simulink model "FMtest"  (R2021a)
settings: Solver=VariableStepAuto  StartTime=0.0  StopTime=3  RelTol=1e-3
undefined symbols (not defined in the file or in its folder): National_Instruments, PCIe
libraries: sldrtlib x4
settings Model: Creator=simmo536  LastModifiedBy=simmo536

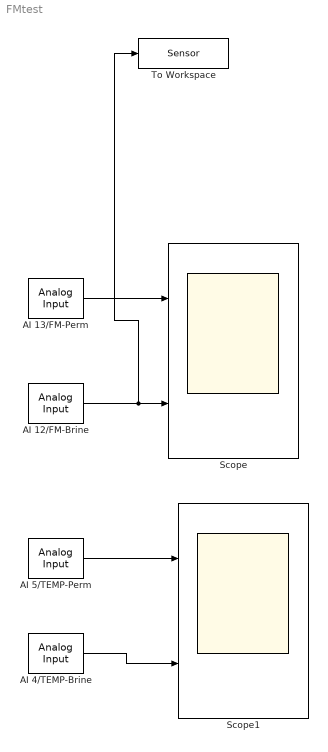
== system FMtest ==
  AI 12/FM-Brine : sldrtlib/Analog Input  SampleTime=0.01  MaxMissedTicks=inf  ShowMissedTicks=off  YieldWhenWaiting=off  DrvName=National_Instruments/PCIe-6343  DrvAddress=4294967295  DrvOptions=[0 0 0 0 0 0 0]  Channels=13  RangeMode=1  VoltRange=1  DataType=2
      settings: AttributesFormatString=National Instruments\nPCIe-6343 [auto]
  AI 13/FM-Perm : sldrtlib/Analog Input  SampleTime=0.01  MaxMissedTicks=inf  ShowMissedTicks=off  YieldWhenWaiting=off  DrvName=National_Instruments/PCIe-6343  DrvAddress=4294967295  DrvOptions=[0 0 0 0 0 0 0]  Channels=14  RangeMode=1  VoltRange=1  DataType=2
      settings: AttributesFormatString=National Instruments\nPCIe-6343 [auto]
  AI 4/TEMP-Brine : sldrtlib/Analog Input  SampleTime=0.01  MaxMissedTicks=inf  ShowMissedTicks=off  YieldWhenWaiting=on  DrvName=National_Instruments/PCIe-6343  DrvAddress=4294967295  DrvOptions=[0 0 0 0 0 0 0]  Channels=5  RangeMode=1  VoltRange=1  DataType=2
      settings: AttributesFormatString=National Instruments\nPCIe-6343 [auto]
  AI 5/TEMP-Perm : sldrtlib/Analog Input  SampleTime=0.01  MaxMissedTicks=inf  ShowMissedTicks=off  YieldWhenWaiting=on  DrvName=National_Instruments/PCIe-6343  DrvAddress=4294967295  DrvOptions=[0 0 0 0 0 0 0]  Channels=6  RangeMode=1  VoltRange=1  DataType=2
      settings: AttributesFormatString=National Instruments\nPCIe-6343 [auto]
  Scope : Scope  NumInputPorts=2
  Scope1 : Scope  NumInputPorts=2
  To Workspace : ToWorkspace  VariableName=Sensor  SaveFormat=Timeseries  SampleTime=-1
  wires:
  AI 13/FM-Perm/1 -> Scope/1
  AI 12/FM-Brine/1 -> To Workspace/1, Scope/2
  AI 4/TEMP-Brine/1 -> Scope1/2
  AI 5/TEMP-Perm/1 -> Scope1/1
